simulink model "project"  (Simulink 7.6)
settings: Solver=ode45  StartTime=0.0  StopTime=10.0  RelTol=1e-3
undefined symbols (not defined in the file): des_attributefunction_support, des_figposition
libraries: simeventsgenerators1 x15, simeventssink1 x13, simeventsattributes2 x11, simeventstranslate1 x4, simeventsrouting1 x3, simeventsserver1 x1
settings Model: Creator=Tima  ModifiedByFormat=Tima  LastModifiedBy=Tima
settings SimEventsCC: propDiagAttribOutput=1  propDiagFcnCallOutput=1  propDiagStatOutput=0

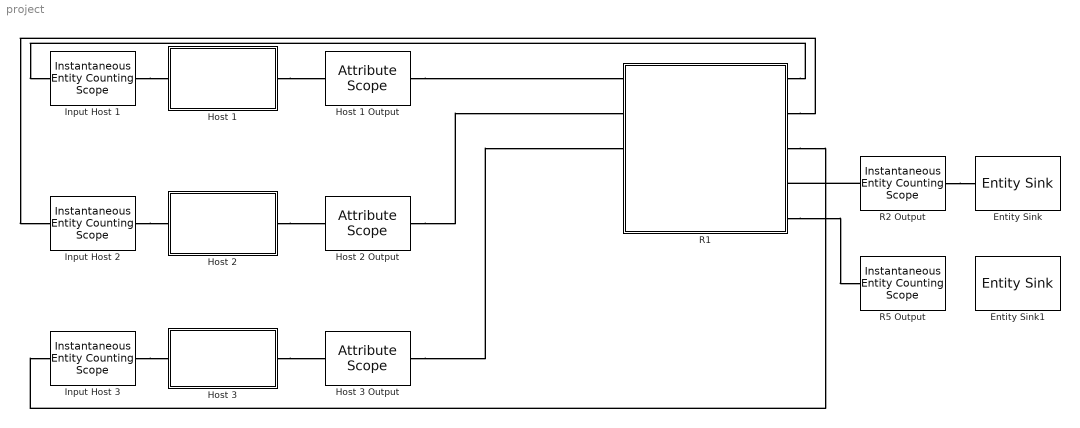
== system project ==
  Entity Sink : simeventssink1/Entity Sink  SystemSampleTime=-1  AvailableForArrivals=on  StatNumberArrived=Off
  Entity Sink1 : simeventssink1/Entity Sink  SystemSampleTime=-1  AvailableForArrivals=on  StatNumberArrived=Off
  Host 1 : Subsystem
  Host 1 Output : simeventssink1/Attribute Scope  SystemSampleTime=-1  PlotType=Stair  InputType=Attribute  NumInputs=1  AttributeNameY=dest  XInputOptionSignal=Event time  XInputOptionEntity=Event time  AttributeNameX=Count  EnableEntityOutport=on  XMin=0  XMax=10  XLimitExceededOption=Stretch axis limits  YLimitExceededOption=Stretch axis limits  AxisGrid=on  AxisLegend=off  LineDisables=""  LineColors=b  LineStyles=-  LineMarkers=.  OpenScopeAtSimStart=on  Title=""  YLabel=""  XLabel=Time  FigurePosition=des_figposition([5 25 25 25])  AxisZoom=off  DataStoreOption=Limited  DataPointsLimit=10000  StatNumberArrived=Off  ShowCountPlotted=off  ShowToolbar=on
      settings: YMin=0  YMax=10
  Host 2 : Subsystem
  Host 2 Output : simeventssink1/Attribute Scope  SystemSampleTime=-1  PlotType=Stair  InputType=Attribute  NumInputs=1  AttributeNameY=dest  XInputOptionSignal=Event time  XInputOptionEntity=Event time  AttributeNameX=Count  EnableEntityOutport=on  XMin=0  XMax=10  XLimitExceededOption=Stretch axis limits  YLimitExceededOption=Stretch axis limits  AxisGrid=on  AxisLegend=off  LineDisables=""  LineColors=b  LineStyles=-  LineMarkers=.  OpenScopeAtSimStart=on  Title=""  YLabel=""  XLabel=Time  FigurePosition=des_figposition([5 25 25 25])  AxisZoom=off  DataStoreOption=Limited  DataPointsLimit=10000  StatNumberArrived=Off  ShowCountPlotted=off  ShowToolbar=on
      settings: YMin=0  YMax=10
  Host 3 : Subsystem
  Host 3 Output : simeventssink1/Attribute Scope  SystemSampleTime=-1  PlotType=Stair  InputType=Attribute  NumInputs=1  AttributeNameY=dest  XInputOptionSignal=Event time  XInputOptionEntity=Event time  AttributeNameX=Count  EnableEntityOutport=on  XMin=0  XMax=10  XLimitExceededOption=Stretch axis limits  YLimitExceededOption=Stretch axis limits  AxisGrid=on  AxisLegend=off  LineDisables=""  LineColors=b  LineStyles=-  LineMarkers=.  OpenScopeAtSimStart=on  Title=""  YLabel=""  XLabel=Time  FigurePosition=des_figposition([5 25 25 25])  AxisZoom=off  DataStoreOption=Limited  DataPointsLimit=10000  StatNumberArrived=Off  ShowCountPlotted=off  ShowToolbar=on
      settings: YMin=0  YMax=10
  Input Host 1 : simeventssink1/Instantaneous Entity Counting Scope  SystemSampleTime=-1  PlotType=Instantaneous entity counting  InputType=Attribute  NumInputs=1  AttributeNameY=Count  XInputOptionSignal=Event time  XInputOptionEntity=Event time  AttributeNameX=Count  EnableEntityOutport=on  XMin=0  XMax=10  XLimitExceededOption=Stretch axis limits  YLimitExceededOption=Stretch axis limits  AxisGrid=on  AxisLegend=off  LineDisables=""  LineColors=b  LineStyles=-  LineMarkers=.  OpenScopeAtSimStart=on  Title=""  YLabel=Number of Entities  XLabel=Time  FigurePosition=des_figposition([5 25 25 25])  AxisZoom=off  DataStoreOption=Limited  DataPointsLimit=10000  StatNumberArrived=Off  ShowCountPlotted=off  ShowToolbar=on
      settings: YMin=0  YMax=10
  Input Host 2 : simeventssink1/Instantaneous Entity Counting Scope  SystemSampleTime=-1  PlotType=Instantaneous entity counting  InputType=Attribute  NumInputs=1  AttributeNameY=Count  XInputOptionSignal=Event time  XInputOptionEntity=Event time  AttributeNameX=Count  EnableEntityOutport=on  XMin=0  XMax=10  XLimitExceededOption=Stretch axis limits  YLimitExceededOption=Stretch axis limits  AxisGrid=on  AxisLegend=off  LineDisables=""  LineColors=b  LineStyles=-  LineMarkers=.  OpenScopeAtSimStart=on  Title=""  YLabel=Number of Entities  XLabel=Time  FigurePosition=des_figposition([5 25 25 25])  AxisZoom=off  DataStoreOption=Limited  DataPointsLimit=10000  StatNumberArrived=Off  ShowCountPlotted=off  ShowToolbar=on
      settings: YMin=0  YMax=10
  Input Host 3 : simeventssink1/Instantaneous Entity Counting Scope  SystemSampleTime=-1  PlotType=Instantaneous entity counting  InputType=Attribute  NumInputs=1  AttributeNameY=Count  XInputOptionSignal=Event time  XInputOptionEntity=Event time  AttributeNameX=Count  EnableEntityOutport=on  XMin=0  XMax=10  XLimitExceededOption=Stretch axis limits  YLimitExceededOption=Stretch axis limits  AxisGrid=on  AxisLegend=off  LineDisables=""  LineColors=b  LineStyles=-  LineMarkers=.  OpenScopeAtSimStart=on  Title=""  YLabel=Number of Entities  XLabel=Time  FigurePosition=des_figposition([5 25 25 25])  AxisZoom=off  DataStoreOption=Limited  DataPointsLimit=10000  StatNumberArrived=Off  ShowCountPlotted=off  ShowToolbar=on
      settings: YMin=0  YMax=10
  R1 : Subsystem
  R2 Output : simeventssink1/Instantaneous Entity Counting Scope  SystemSampleTime=-1  PlotType=Instantaneous entity counting  InputType=Attribute  NumInputs=1  AttributeNameY=Count  XInputOptionSignal=Event time  XInputOptionEntity=Event time  AttributeNameX=Count  EnableEntityOutport=on  XMin=0  XMax=10  XLimitExceededOption=Stretch axis limits  YLimitExceededOption=Stretch axis limits  AxisGrid=on  AxisLegend=off  LineDisables=""  LineColors=b  LineStyles=-  LineMarkers=.  OpenScopeAtSimStart=on  Title=""  YLabel=Number of Entities  XLabel=Time  FigurePosition=des_figposition([5 25 25 25])  AxisZoom=off  DataStoreOption=Limited  DataPointsLimit=10000  StatNumberArrived=Off  ShowCountPlotted=off  ShowToolbar=on
      settings: YMin=0  YMax=10
  R5 Output : simeventssink1/Instantaneous Entity Counting Scope  SystemSampleTime=-1  PlotType=Instantaneous entity counting  InputType=Attribute  NumInputs=1  AttributeNameY=Count  XInputOptionSignal=Event time  XInputOptionEntity=Event time  AttributeNameX=Count  EnableEntityOutport=on  XMin=0  XMax=10  XLimitExceededOption=Stretch axis limits  YLimitExceededOption=Stretch axis limits  AxisGrid=on  AxisLegend=off  LineDisables=""  LineColors=b  LineStyles=-  LineMarkers=.  OpenScopeAtSimStart=on  Title=""  YLabel=Number of Entities  XLabel=Time  FigurePosition=des_figposition([5 25 25 25])  AxisZoom=off  DataStoreOption=Limited  DataPointsLimit=10000  StatNumberArrived=Off  ShowCountPlotted=off  ShowToolbar=on
      settings: YMin=0  YMax=10
  connections:
  Host 1/RConn1 -- Host 1 Output/LConn1
  Host 1 Output/RConn1 -- R1/LConn1
  Host 2/RConn1 -- Host 2 Output/LConn1
  Host 2 Output/RConn1 -- R1/LConn2
  Host 3/RConn1 -- Host 3 Output/LConn1
  Host 3 Output/RConn1 -- R1/LConn3
  Input Host 3/RConn1 -- Host 3/LConn1
  R1/RConn3 -- Input Host 3/LConn1
  R1/RConn1 -- Input Host 1/LConn1
  Input Host 1/RConn1 -- Host 1/LConn1
  R1/RConn2 -- Input Host 2/LConn1
  Input Host 2/RConn1 -- Host 2/LConn1
  R2 Output/LConn1 -- R1/RConn4
  R2 Output/RConn1 -- Entity Sink/LConn1
  R1/RConn5 -- R5 Output/LConn1

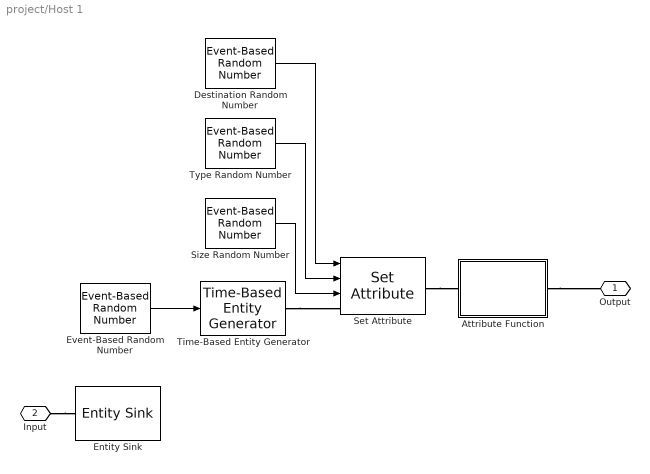
== system project/Host 1 ==
  Attribute Function : Subsystem  LoadFcn=des_attributefunction_support(gcb,'LoadFcn');  StartFcn=des_attributefunction_support(gcb,'StartFcn');  mask(Attribute Function){OutputNamePrefix=out_}
      mask prompts: OutputNamePrefix "Prefix name"
      settings: CopyFcn=des_attributefunction_support(gcb,'CopyFcn');  OpenFcn=des_attributefunction_support(gcb,'OpenFcn');  ErrorFcn=des_error_redirect
      mask Help: helpview(simeventsbhelp('attributefunction'))
      mask Display: image(des_iconLoad('attribFunction.jpg'),'center');
  Destination Random Number : simeventsgenerators1/Signal Generators/Event-Based Random Number  SystemSampleTime=-1  distribution=Discrete uniform  meanExp=1  minUnif=1  maxUnif=1  pOneBern=0.25  pSuccessBino=0.5  numTrialBino=1  meanNorm=0  stdNorm=1  minTri=1  maxTri=3  modeTri=2  thresholdLogn=0  scaleLogn=1  shapeLogn=1  pSuccessGeo=0.5  meanPoiss=1  thresholdLogl=0  scaleLogl=1  thresholdGam=0  scaleGam=1  shapeGam=1  minBeta=0  maxBeta=1  shape1Beta=1  shape2Beta=1  minUnid=1  maxUnid=6  numValueUnid=6  thresholdWbl=0  scaleWbl=1  shapeWbl=1  valueVecCont=[0 1]  cdfVecCont=[0 1]  valueVecDisc=[0 1]  probVecDisc=[0.5 0.5]  seed=897465  IsProcessed=on  isConnected=1
  Entity Sink : simeventssink1/Entity Sink  SystemSampleTime=-1  AvailableForArrivals=on  StatNumberArrived=Off
  Event-Based Random Number : simeventsgenerators1/Signal Generators/Event-Based Random Number  SystemSampleTime=-1  distribution=Poisson  meanExp=1  minUnif=1  maxUnif=1  pOneBern=0.25  pSuccessBino=0.5  numTrialBino=1  meanNorm=0  stdNorm=1  minTri=1  maxTri=3  modeTri=2  thresholdLogn=0  scaleLogn=1  shapeLogn=1  pSuccessGeo=0.5  meanPoiss=1  thresholdLogl=0  scaleLogl=1  thresholdGam=0  scaleGam=1  shapeGam=1  minBeta=0  maxBeta=1  shape1Beta=1  shape2Beta=1  minUnid=0  maxUnid=1  numValueUnid=2  thresholdWbl=0  scaleWbl=1  shapeWbl=1  valueVecCont=[0 1]  cdfVecCont=[0 1]  valueVecDisc=[0 1]  probVecDisc=[0.5 0.5]  seed=54353  IsProcessed=on  isConnected=1
  Set Attribute : simeventsattributes2/Set Attribute  DialogController=des_ddg_create  DialogControllerArgs=DataTag9  SystemSampleTime=-1  AttributeFrom=Signal port|Signal port|Signal port  AttributeName=dest|type|size  AttributeTreatAsVector=1|1|1  AttributeValue=1|1|1  AttributeCreate=on  StatNumberDeparted=Off  EvaluatedAttributeValue={[];[];[]}
  Size Random Number : simeventsgenerators1/Signal Generators/Event-Based Random Number  SystemSampleTime=-1  distribution=Discrete uniform  meanExp=1  minUnif=1  maxUnif=1  pOneBern=0.25  pSuccessBino=0.5  numTrialBino=1  meanNorm=0  stdNorm=1  minTri=1  maxTri=3  modeTri=2  thresholdLogn=0  scaleLogn=1  shapeLogn=1  pSuccessGeo=0.5  meanPoiss=1  thresholdLogl=0  scaleLogl=1  thresholdGam=0  scaleGam=1  shapeGam=1  minBeta=0  maxBeta=1  shape1Beta=1  shape2Beta=1  minUnid=1  maxUnid=2  numValueUnid=2  thresholdWbl=0  scaleWbl=1  shapeWbl=1  valueVecCont=[0 1]  cdfVecCont=[0 1]  valueVecDisc=[0 1]  probVecDisc=[0.5 0.5]  seed=79846  IsProcessed=on  isConnected=1
  Time-Based Entity Generator : simeventsgenerators1/Entity Generators/Time-Based Entity Generator  DialogController=des_ddg_create  DialogControllerArgs=DataTag11  SystemSampleTime=-1  GenerateEntitiesUpon=Intergeneration time from port t  Distribution=Constant  Minimum=0  Maximum=1  Mean=1  InitialSeed=12345  Period=1  PriorityEntityGeneration=300  GenerateEntityAtSimulationStart=on  ResponseWhenBlocked=Pause generation  ResponseWhenUnblocked=Immediate restart  EntityType=Blank  StatNumberDeparted=Off  StatPendingEntity=Off  StatAverageIntergenerationTime=Off
  Type Random Number : simeventsgenerators1/Signal Generators/Event-Based Random Number  SystemSampleTime=-1  distribution=Discrete uniform  meanExp=1  minUnif=1  maxUnif=1  pOneBern=0.25  pSuccessBino=0.5  numTrialBino=1  meanNorm=0  stdNorm=1  minTri=1  maxTri=3  modeTri=2  thresholdLogn=0  scaleLogn=1  shapeLogn=1  pSuccessGeo=0.5  meanPoiss=1  thresholdLogl=0  scaleLogl=1  thresholdGam=0  scaleGam=1  shapeGam=1  minBeta=0  maxBeta=1  shape1Beta=1  shape2Beta=1  minUnid=1  maxUnid=2  numValueUnid=2  thresholdWbl=0  scaleWbl=1  shapeWbl=1  valueVecCont=[0 1]  cdfVecCont=[0 1]  valueVecDisc=[0 1]  probVecDisc=[0.5 0.5]  seed=7865687  IsProcessed=on  isConnected=1
  Output : PMIOPort  Port=1  Side=Right
  Input : PMIOPort  Port=2  Side=Left
  wires:
  Event-Based Random Number/1 -> Time-Based Entity Generator/1
  Destination Random Number/1 -> Set Attribute/1
  Type Random Number/1 -> Set Attribute/2
  Size Random Number/1 -> Set Attribute/3
  connections:
  Set Attribute/RConn1 -- Attribute Function/LConn1
  Time-Based Entity Generator/RConn1 -- Set Attribute/LConn1
  Input/RConn1 -- Entity Sink/LConn1
  Attribute Function/RConn1 -- Output/RConn1

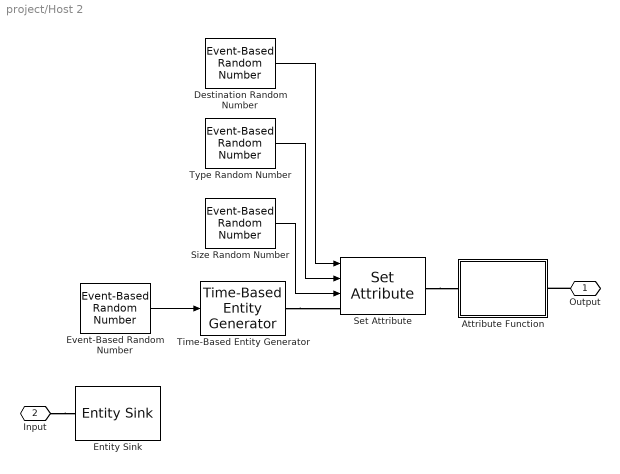
== system project/Host 2 ==
  Attribute Function : Subsystem  LoadFcn=des_attributefunction_support(gcb,'LoadFcn');  StartFcn=des_attributefunction_support(gcb,'StartFcn');  mask(Attribute Function){OutputNamePrefix=out_}
      mask prompts: OutputNamePrefix "Prefix name"
      settings: CopyFcn=des_attributefunction_support(gcb,'CopyFcn');  OpenFcn=des_attributefunction_support(gcb,'OpenFcn');  ErrorFcn=des_error_redirect
      mask Help: helpview(simeventsbhelp('attributefunction'))
      mask Display: image(des_iconLoad('attribFunction.jpg'),'center');
  Destination Random Number : simeventsgenerators1/Signal Generators/Event-Based Random Number  SystemSampleTime=-1  distribution=Discrete uniform  meanExp=1  minUnif=1  maxUnif=1  pOneBern=0.25  pSuccessBino=0.5  numTrialBino=1  meanNorm=0  stdNorm=1  minTri=1  maxTri=3  modeTri=2  thresholdLogn=0  scaleLogn=1  shapeLogn=1  pSuccessGeo=0.5  meanPoiss=1  thresholdLogl=0  scaleLogl=1  thresholdGam=0  scaleGam=1  shapeGam=1  minBeta=0  maxBeta=1  shape1Beta=1  shape2Beta=1  minUnid=1  maxUnid=6  numValueUnid=6  thresholdWbl=0  scaleWbl=1  shapeWbl=1  valueVecCont=[0 1]  cdfVecCont=[0 1]  valueVecDisc=[0 1]  probVecDisc=[0.5 0.5]  seed=8698465  IsProcessed=on  isConnected=1
  Entity Sink : simeventssink1/Entity Sink  SystemSampleTime=-1  AvailableForArrivals=on  StatNumberArrived=Off
  Event-Based Random Number : simeventsgenerators1/Signal Generators/Event-Based Random Number  SystemSampleTime=-1  distribution=Poisson  meanExp=1  minUnif=1  maxUnif=1  pOneBern=0.25  pSuccessBino=0.5  numTrialBino=1  meanNorm=0  stdNorm=1  minTri=1  maxTri=3  modeTri=2  thresholdLogn=0  scaleLogn=1  shapeLogn=1  pSuccessGeo=0.5  meanPoiss=1  thresholdLogl=0  scaleLogl=1  thresholdGam=0  scaleGam=1  shapeGam=1  minBeta=0  maxBeta=1  shape1Beta=1  shape2Beta=1  minUnid=0  maxUnid=1  numValueUnid=2  thresholdWbl=0  scaleWbl=1  shapeWbl=1  valueVecCont=[0 1]  cdfVecCont=[0 1]  valueVecDisc=[0 1]  probVecDisc=[0.5 0.5]  seed=43643  IsProcessed=on  isConnected=1
  Set Attribute : simeventsattributes2/Set Attribute  DialogController=des_ddg_create  DialogControllerArgs=DataTag20  SystemSampleTime=-1  AttributeFrom=Signal port|Signal port|Signal port  AttributeName=dest|type|size  AttributeTreatAsVector=1|1|1  AttributeValue=1|1|1  AttributeCreate=on  StatNumberDeparted=Off  EvaluatedAttributeValue={[];[];[]}
  Size Random Number : simeventsgenerators1/Signal Generators/Event-Based Random Number  SystemSampleTime=-1  distribution=Discrete uniform  meanExp=1  minUnif=1  maxUnif=1  pOneBern=0.25  pSuccessBino=0.5  numTrialBino=1  meanNorm=0  stdNorm=1  minTri=1  maxTri=3  modeTri=2  thresholdLogn=0  scaleLogn=1  shapeLogn=1  pSuccessGeo=0.5  meanPoiss=1  thresholdLogl=0  scaleLogl=1  thresholdGam=0  scaleGam=1  shapeGam=1  minBeta=0  maxBeta=1  shape1Beta=1  shape2Beta=1  minUnid=1  maxUnid=2  numValueUnid=2  thresholdWbl=0  scaleWbl=1  shapeWbl=1  valueVecCont=[0 1]  cdfVecCont=[0 1]  valueVecDisc=[0 1]  probVecDisc=[0.5 0.5]  seed=987654  IsProcessed=on  isConnected=1
  Time-Based Entity Generator : simeventsgenerators1/Entity Generators/Time-Based Entity Generator  DialogController=des_ddg_create  DialogControllerArgs=DataTag22  SystemSampleTime=-1  GenerateEntitiesUpon=Intergeneration time from port t  Distribution=Constant  Minimum=0  Maximum=1  Mean=1  InitialSeed=12345  Period=1  PriorityEntityGeneration=300  GenerateEntityAtSimulationStart=on  ResponseWhenBlocked=Pause generation  ResponseWhenUnblocked=Immediate restart  EntityType=Blank  StatNumberDeparted=Off  StatPendingEntity=Off  StatAverageIntergenerationTime=Off
  Type Random Number : simeventsgenerators1/Signal Generators/Event-Based Random Number  SystemSampleTime=-1  distribution=Discrete uniform  meanExp=1  minUnif=1  maxUnif=1  pOneBern=0.25  pSuccessBino=0.5  numTrialBino=1  meanNorm=0  stdNorm=1  minTri=1  maxTri=3  modeTri=2  thresholdLogn=0  scaleLogn=1  shapeLogn=1  pSuccessGeo=0.5  meanPoiss=1  thresholdLogl=0  scaleLogl=1  thresholdGam=0  scaleGam=1  shapeGam=1  minBeta=0  maxBeta=1  shape1Beta=1  shape2Beta=1  minUnid=1  maxUnid=2  numValueUnid=2  thresholdWbl=0  scaleWbl=1  shapeWbl=1  valueVecCont=[0 1]  cdfVecCont=[0 1]  valueVecDisc=[0 1]  probVecDisc=[0.5 0.5]  seed=869846  IsProcessed=on  isConnected=1
  Output : PMIOPort  Port=1  Side=Right
  Input : PMIOPort  Port=2  Side=Left
  wires:
  Size Random Number/1 -> Set Attribute/3
  Type Random Number/1 -> Set Attribute/2
  Destination Random Number/1 -> Set Attribute/1
  Event-Based Random Number/1 -> Time-Based Entity Generator/1
  connections:
  Input/RConn1 -- Entity Sink/LConn1
  Output/RConn1 -- Attribute Function/RConn1
  Time-Based Entity Generator/RConn1 -- Set Attribute/LConn1
  Set Attribute/RConn1 -- Attribute Function/LConn1

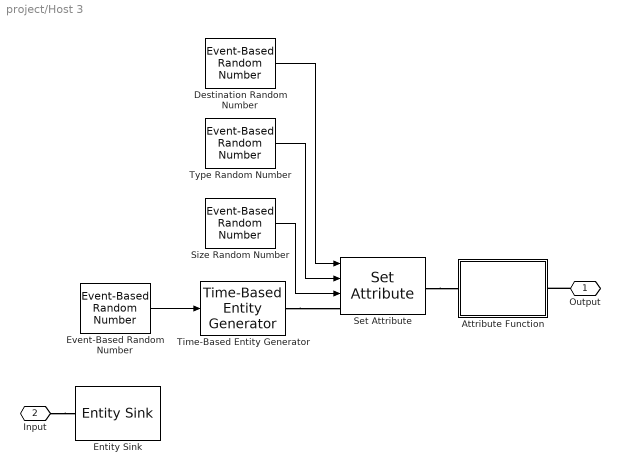
== system project/Host 3 ==
  Attribute Function : Subsystem  LoadFcn=des_attributefunction_support(gcb,'LoadFcn');  StartFcn=des_attributefunction_support(gcb,'StartFcn');  mask(Attribute Function){OutputNamePrefix=out_}
      mask prompts: OutputNamePrefix "Prefix name"
      settings: CopyFcn=des_attributefunction_support(gcb,'CopyFcn');  OpenFcn=des_attributefunction_support(gcb,'OpenFcn');  ErrorFcn=des_error_redirect
      mask Help: helpview(simeventsbhelp('attributefunction'))
      mask Display: image(des_iconLoad('attribFunction.jpg'),'center');
  Destination Random Number : simeventsgenerators1/Signal Generators/Event-Based Random Number  SystemSampleTime=-1  distribution=Discrete uniform  meanExp=1  minUnif=1  maxUnif=1  pOneBern=0.25  pSuccessBino=0.5  numTrialBino=1  meanNorm=0  stdNorm=1  minTri=1  maxTri=3  modeTri=2  thresholdLogn=0  scaleLogn=1  shapeLogn=1  pSuccessGeo=0.5  meanPoiss=1  thresholdLogl=0  scaleLogl=1  thresholdGam=0  scaleGam=1  shapeGam=1  minBeta=0  maxBeta=1  shape1Beta=1  shape2Beta=1  minUnid=1  maxUnid=6  numValueUnid=6  thresholdWbl=0  scaleWbl=1  shapeWbl=1  valueVecCont=[0 1]  cdfVecCont=[0 1]  valueVecDisc=[0 1]  probVecDisc=[0.5 0.5]  seed=964  IsProcessed=on  isConnected=1
  Entity Sink : simeventssink1/Entity Sink  SystemSampleTime=-1  AvailableForArrivals=on  StatNumberArrived=Off
  Event-Based Random Number : simeventsgenerators1/Signal Generators/Event-Based Random Number  SystemSampleTime=-1  distribution=Poisson  meanExp=1  minUnif=1  maxUnif=1  pOneBern=0.25  pSuccessBino=0.5  numTrialBino=1  meanNorm=0  stdNorm=1  minTri=1  maxTri=3  modeTri=2  thresholdLogn=0  scaleLogn=1  shapeLogn=1  pSuccessGeo=0.5  meanPoiss=1  thresholdLogl=0  scaleLogl=1  thresholdGam=0  scaleGam=1  shapeGam=1  minBeta=0  maxBeta=1  shape1Beta=1  shape2Beta=1  minUnid=0  maxUnid=1  numValueUnid=2  thresholdWbl=0  scaleWbl=1  shapeWbl=1  valueVecCont=[0 1]  cdfVecCont=[0 1]  valueVecDisc=[0 1]  probVecDisc=[0.5 0.5]  seed=12345  IsProcessed=on  isConnected=1
  Set Attribute : simeventsattributes2/Set Attribute  DialogController=des_ddg_create  DialogControllerArgs=DataTag31  SystemSampleTime=-1  AttributeFrom=Signal port|Signal port|Signal port  AttributeName=dest|type|size  AttributeTreatAsVector=1|1|1  AttributeValue=1|1|1  AttributeCreate=on  StatNumberDeparted=Off  EvaluatedAttributeValue={[];[];[]}
  Size Random Number : simeventsgenerators1/Signal Generators/Event-Based Random Number  SystemSampleTime=-1  distribution=Discrete uniform  meanExp=1  minUnif=1  maxUnif=1  pOneBern=0.25  pSuccessBino=0.5  numTrialBino=1  meanNorm=0  stdNorm=1  minTri=1  maxTri=3  modeTri=2  thresholdLogn=0  scaleLogn=1  shapeLogn=1  pSuccessGeo=0.5  meanPoiss=1  thresholdLogl=0  scaleLogl=1  thresholdGam=0  scaleGam=1  shapeGam=1  minBeta=0  maxBeta=1  shape1Beta=1  shape2Beta=1  minUnid=1  maxUnid=2  numValueUnid=2  thresholdWbl=0  scaleWbl=1  shapeWbl=1  valueVecCont=[0 1]  cdfVecCont=[0 1]  valueVecDisc=[0 1]  probVecDisc=[0.5 0.5]  seed=13245  IsProcessed=on  isConnected=1
  Time-Based Entity Generator : simeventsgenerators1/Entity Generators/Time-Based Entity Generator  DialogController=des_ddg_create  DialogControllerArgs=DataTag33  SystemSampleTime=-1  GenerateEntitiesUpon=Intergeneration time from port t  Distribution=Constant  Minimum=0  Maximum=1  Mean=1  InitialSeed=12345  Period=1  PriorityEntityGeneration=300  GenerateEntityAtSimulationStart=on  ResponseWhenBlocked=Pause generation  ResponseWhenUnblocked=Immediate restart  EntityType=Blank  StatNumberDeparted=Off  StatPendingEntity=Off  StatAverageIntergenerationTime=Off
  Type Random Number : simeventsgenerators1/Signal Generators/Event-Based Random Number  SystemSampleTime=-1  distribution=Discrete uniform  meanExp=1  minUnif=1  maxUnif=1  pOneBern=0.25  pSuccessBino=0.5  numTrialBino=1  meanNorm=0  stdNorm=1  minTri=1  maxTri=3  modeTri=2  thresholdLogn=0  scaleLogn=1  shapeLogn=1  pSuccessGeo=0.5  meanPoiss=1  thresholdLogl=0  scaleLogl=1  thresholdGam=0  scaleGam=1  shapeGam=1  minBeta=0  maxBeta=1  shape1Beta=1  shape2Beta=1  minUnid=1  maxUnid=2  numValueUnid=2  thresholdWbl=0  scaleWbl=1  shapeWbl=1  valueVecCont=[0 1]  cdfVecCont=[0 1]  valueVecDisc=[0 1]  probVecDisc=[0.5 0.5]  seed=6745  IsProcessed=on  isConnected=1
  Output : PMIOPort  Port=1  Side=Right
  Input : PMIOPort  Port=2  Side=Left
  wires:
  Event-Based Random Number/1 -> Time-Based Entity Generator/1
  Destination Random Number/1 -> Set Attribute/1
  Type Random Number/1 -> Set Attribute/2
  Size Random Number/1 -> Set Attribute/3
  connections:
  Set Attribute/RConn1 -- Attribute Function/LConn1
  Time-Based Entity Generator/RConn1 -- Set Attribute/LConn1
  Output/RConn1 -- Attribute Function/RConn1
  Input/RConn1 -- Entity Sink/LConn1

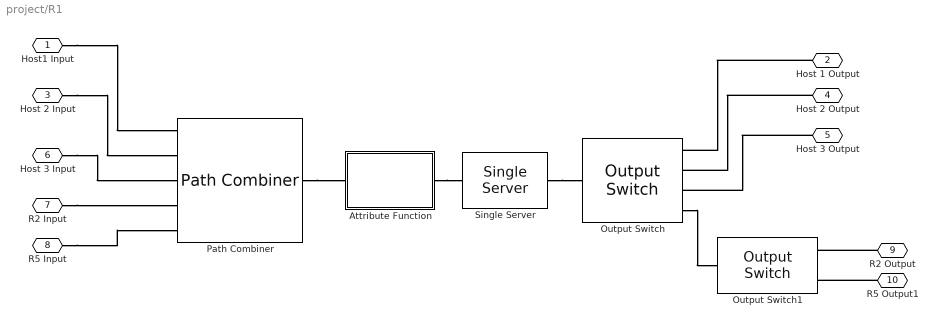
== system project/R1 ==
  Attribute Function : Subsystem  LoadFcn=des_attributefunction_support(gcb,'LoadFcn');  StartFcn=des_attributefunction_support(gcb,'StartFcn');  mask(Attribute Function){OutputNamePrefix=out_}
      mask prompts: OutputNamePrefix "Prefix name"
      settings: CopyFcn=des_attributefunction_support(gcb,'CopyFcn');  OpenFcn=des_attributefunction_support(gcb,'OpenFcn');  ErrorFcn=des_error_redirect
      mask Help: helpview(simeventsbhelp('attributefunction'))
      mask Display: image(des_iconLoad('attribFunction.jpg'),'center');
  Output Switch : simeventsrouting1/Output Switch  SystemSampleTime=-1  NumberOutputPorts=4  SwitchingCriterion=From attribute  InitialSeed=34567  AttributeName=port  InitialConditionsOpt=off  InitialConditions=1  EntityBufferOpt=off  SpecifyEventPriority=off  PriorityOutputSwitchSelectPort=4100  TimeoutPortOpt=off  StatNumberDeparted=Off  StatNumberTimedOut=Off  StatPendingEntity=Off  StatLastDeparturePort=Off  EvaluatedNumPorts=4
  Output Switch1 : simeventsrouting1/Output Switch  SystemSampleTime=-1  NumberOutputPorts=2  SwitchingCriterion=First port that is not blocked  InitialSeed=34567  AttributeName=Attribute1  InitialConditionsOpt=off  InitialConditions=1  EntityBufferOpt=off  SpecifyEventPriority=off  PriorityOutputSwitchSelectPort=4100  TimeoutPortOpt=off  StatNumberDeparted=Off  StatNumberTimedOut=Off  StatPendingEntity=Off  StatLastDeparturePort=Off  EvaluatedNumPorts=2
  Path Combiner : simeventsrouting1/Path Combiner  SystemSampleTime=-1  NumberInputPorts=5  InputPortPrecedence=IN1 port  InitialSeed=45675  SpecifyEventPriority=off  PriorityPathCombinerPortPrecedenceSelection=4100  StatNumberDeparted=Off  StatLastArrivalPort=Off  EvaluatedNumPorts=5
  Single Server : simeventsserver1/Single Server  SystemSampleTime=-1  ServiceTimeFrom=Dialog  ServiceTime=0  AttributeName=ServiceTime  PriorityServiceCompletion=500  PermitPreemption=off  SortingAttributeName=PriorityAttributeName  SortingDirection=Ascending  WriteToAttribute=off  ResidualAttributeName=ResidualServiceTime  CreateAttribute=on  EnableTOPort=off  StatNumberDeparted=Off  StatNumberInBlock=Off  StatNumberPreempted=Off  StatPendingEntity=Off  StatAverageWait=Off  StatUtilization=Off  StatNumberTimedout=Off
  Host1 Input : PMIOPort  Port=1  Side=Left
  Host 1 Output : PMIOPort  Port=2  Side=Right
  Host 2 Input : PMIOPort  Port=3  Side=Left
  Host 2 Output : PMIOPort  Port=4  Side=Right
  Host 3 Output : PMIOPort  Port=5  Side=Right
  Host 3 Input : PMIOPort  Port=6  Side=Left
  R2 Input : PMIOPort  Port=7  Side=Left
  R5 Input : PMIOPort  Port=8  Side=Left
  R2 Output : PMIOPort  Port=9  Side=Right
  R5 Output1 : PMIOPort  Port=10  Side=Right
  connections:
  Path Combiner/RConn1 -- Attribute Function/LConn1
  Host 1 Output/RConn1 -- Output Switch/RConn1
  Host 2 Output/RConn1 -- Output Switch/RConn2
  Host 3 Output/RConn1 -- Output Switch/RConn3
  Host1 Input/RConn1 -- Path Combiner/LConn1
  Host 2 Input/RConn1 -- Path Combiner/LConn2
  Host 3 Input/RConn1 -- Path Combiner/LConn3
  R2 Input/RConn1 -- Path Combiner/LConn4
  R5 Input/RConn1 -- Path Combiner/LConn5
  Output Switch/RConn4 -- Output Switch1/LConn1
  R2 Output/RConn1 -- Output Switch1/RConn1
  R5 Output1/RConn1 -- Output Switch1/RConn2
  Attribute Function/RConn1 -- Single Server/LConn1
  Single Server/RConn1 -- Output Switch/LConn1

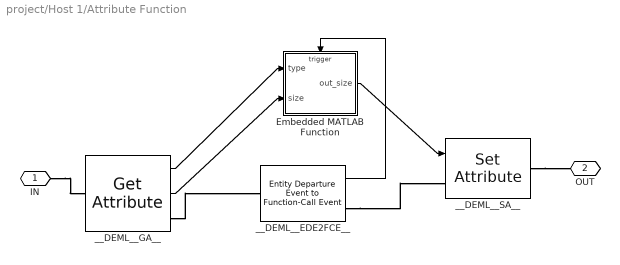
== system project/Host 1/Attribute Function ==
  Embedded MATLAB Function : Stateflow chart  TreatAsAtomicUnit=on
      settings: PropExecContextOutsideSubsystem=on
  __DEML__EDE2FCE__ : simeventstranslate1/Entity Departure Event to Function-Call Event  Priority=1  SystemSampleTime=-1  TimingFunctionCallF1=Before entity departure  EnableE1Port=off  EnableF2Port=off  TimingFunctionCallF2=Before entity departure  EnableE2Port=off  StatNumberDeparted=Off  StatNumberF1Calls=Off  StatNumberF2Calls=Off  IsInsideAFB=on
  __DEML__GA__ : simeventsattributes2/Get Attribute  Priority=1  DialogController=des_ddg_create  DialogControllerArgs=DataTag4  SystemSampleTime=-1  AttributeName=type|size  AttributeMissing=Error|Error  AttributeDefaultValue=1|1  AttributeSendTiming=Before entity departure|Before entity departure  AttributeTreatAsVector=1|1  StatNumberDeparted=Off  EvaluatedDefaultAttributeValue={[];[]}
  __DEML__SA__ : simeventsattributes2/Set Attribute  Priority=1  DialogController=des_ddg_create  DialogControllerArgs=DataTag6  SystemSampleTime=-1  AttributeFrom=Signal port  AttributeName=size  AttributeTreatAsVector=1  AttributeValue=1  AttributeCreate=on  StatNumberDeparted=Off  EvaluatedAttributeValue={[]}
  IN : PMIOPort  Port=1  Side=Left
  OUT : PMIOPort  Port=2  Side=Right
  wires:
  __DEML__EDE2FCE__/1 -> Embedded MATLAB Function/Trigger
  __DEML__GA__/1 -> Embedded MATLAB Function/1(type)
  __DEML__GA__/2 -> Embedded MATLAB Function/2(size)
  Embedded MATLAB Function/1(out_size) -> __DEML__SA__/1
  connections:
  __DEML__SA__/RConn1 -- OUT/RConn1
  IN/RConn1 -- __DEML__GA__/LConn1
  __DEML__GA__/RConn1 -- __DEML__EDE2FCE__/LConn1
  __DEML__EDE2FCE__/RConn1 -- __DEML__SA__/LConn1

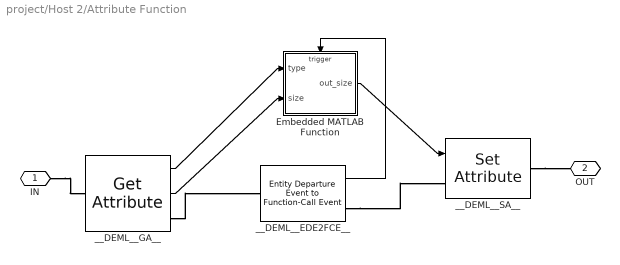
== system project/Host 2/Attribute Function ==
  Embedded MATLAB Function : Stateflow chart  TreatAsAtomicUnit=on
      settings: PropExecContextOutsideSubsystem=on
  __DEML__EDE2FCE__ : simeventstranslate1/Entity Departure Event to Function-Call Event  Priority=1  SystemSampleTime=-1  TimingFunctionCallF1=Before entity departure  EnableE1Port=off  EnableF2Port=off  TimingFunctionCallF2=Before entity departure  EnableE2Port=off  StatNumberDeparted=Off  StatNumberF1Calls=Off  StatNumberF2Calls=Off  IsInsideAFB=on
  __DEML__GA__ : simeventsattributes2/Get Attribute  Priority=1  DialogController=des_ddg_create  DialogControllerArgs=DataTag15  SystemSampleTime=-1  AttributeName=type|size  AttributeMissing=Error|Error  AttributeDefaultValue=1|1  AttributeSendTiming=Before entity departure|Before entity departure  AttributeTreatAsVector=1|1  StatNumberDeparted=Off  EvaluatedDefaultAttributeValue={[];[]}
  __DEML__SA__ : simeventsattributes2/Set Attribute  Priority=1  DialogController=des_ddg_create  DialogControllerArgs=DataTag17  SystemSampleTime=-1  AttributeFrom=Signal port  AttributeName=size  AttributeTreatAsVector=1  AttributeValue=1  AttributeCreate=on  StatNumberDeparted=Off  EvaluatedAttributeValue={[]}
  IN : PMIOPort  Port=1  Side=Left
  OUT : PMIOPort  Port=2  Side=Right
  wires:
  __DEML__EDE2FCE__/1 -> Embedded MATLAB Function/Trigger
  __DEML__GA__/1 -> Embedded MATLAB Function/1(type)
  __DEML__GA__/2 -> Embedded MATLAB Function/2(size)
  Embedded MATLAB Function/1(out_size) -> __DEML__SA__/1
  connections:
  __DEML__EDE2FCE__/RConn1 -- __DEML__SA__/LConn1
  __DEML__GA__/RConn1 -- __DEML__EDE2FCE__/LConn1
  IN/RConn1 -- __DEML__GA__/LConn1
  __DEML__SA__/RConn1 -- OUT/RConn1

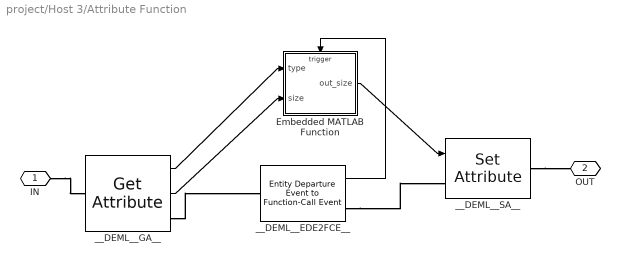
== system project/Host 3/Attribute Function ==
  Embedded MATLAB Function : Stateflow chart  TreatAsAtomicUnit=on
      settings: PropExecContextOutsideSubsystem=on
  __DEML__EDE2FCE__ : simeventstranslate1/Entity Departure Event to Function-Call Event  Priority=1  SystemSampleTime=-1  TimingFunctionCallF1=Before entity departure  EnableE1Port=off  EnableF2Port=off  TimingFunctionCallF2=Before entity departure  EnableE2Port=off  StatNumberDeparted=Off  StatNumberF1Calls=Off  StatNumberF2Calls=Off  IsInsideAFB=on
  __DEML__GA__ : simeventsattributes2/Get Attribute  Priority=1  DialogController=des_ddg_create  DialogControllerArgs=DataTag26  SystemSampleTime=-1  AttributeName=type|size  AttributeMissing=Error|Error  AttributeDefaultValue=1|1  AttributeSendTiming=Before entity departure|Before entity departure  AttributeTreatAsVector=1|1  StatNumberDeparted=Off  EvaluatedDefaultAttributeValue={[];[]}
  __DEML__SA__ : simeventsattributes2/Set Attribute  Priority=1  DialogController=des_ddg_create  DialogControllerArgs=DataTag28  SystemSampleTime=-1  AttributeFrom=Signal port  AttributeName=size  AttributeTreatAsVector=1  AttributeValue=1  AttributeCreate=on  StatNumberDeparted=Off  EvaluatedAttributeValue={[]}
  IN : PMIOPort  Port=1  Side=Left
  OUT : PMIOPort  Port=2  Side=Right
  wires:
  __DEML__EDE2FCE__/1 -> Embedded MATLAB Function/Trigger
  __DEML__GA__/1 -> Embedded MATLAB Function/1(type)
  __DEML__GA__/2 -> Embedded MATLAB Function/2(size)
  Embedded MATLAB Function/1(out_size) -> __DEML__SA__/1
  connections:
  __DEML__SA__/RConn1 -- OUT/RConn1
  IN/RConn1 -- __DEML__GA__/LConn1
  __DEML__GA__/RConn1 -- __DEML__EDE2FCE__/LConn1
  __DEML__EDE2FCE__/RConn1 -- __DEML__SA__/LConn1

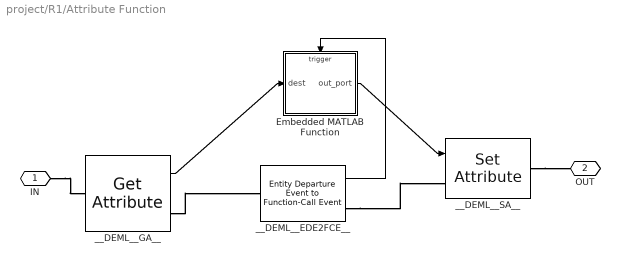
== system project/R1/Attribute Function ==
  Embedded MATLAB Function : Stateflow chart  TreatAsAtomicUnit=on
      settings: PropExecContextOutsideSubsystem=on
  __DEML__EDE2FCE__ : simeventstranslate1/Entity Departure Event to Function-Call Event  Priority=1  SystemSampleTime=-1  TimingFunctionCallF1=Before entity departure  EnableE1Port=off  EnableF2Port=off  TimingFunctionCallF2=Before entity departure  EnableE2Port=off  StatNumberDeparted=Off  StatNumberF1Calls=Off  StatNumberF2Calls=Off  IsInsideAFB=on
  __DEML__GA__ : simeventsattributes2/Get Attribute  Priority=1  DialogController=des_ddg_create  DialogControllerArgs=DataTag40  SystemSampleTime=-1  AttributeName=dest  AttributeMissing=Error  AttributeDefaultValue=1  AttributeSendTiming=Before entity departure  AttributeTreatAsVector=1  StatNumberDeparted=Off  EvaluatedDefaultAttributeValue={[]}
  __DEML__SA__ : simeventsattributes2/Set Attribute  Priority=1  DialogController=des_ddg_create  DialogControllerArgs=DataTag42  SystemSampleTime=-1  AttributeFrom=Signal port  AttributeName=port  AttributeTreatAsVector=1  AttributeValue=1  AttributeCreate=on  StatNumberDeparted=Off  EvaluatedAttributeValue={[]}
  IN : PMIOPort  Port=1  Side=Left
  OUT : PMIOPort  Port=2  Side=Right
  wires:
  __DEML__EDE2FCE__/1 -> Embedded MATLAB Function/Trigger
  __DEML__GA__/1 -> Embedded MATLAB Function/1(dest)
  Embedded MATLAB Function/1(out_port) -> __DEML__SA__/1
  connections:
  __DEML__SA__/RConn1 -- OUT/RConn1
  IN/RConn1 -- __DEML__GA__/LConn1
  __DEML__GA__/RConn1 -- __DEML__EDE2FCE__/LConn1
  __DEML__EDE2FCE__/RConn1 -- __DEML__SA__/LConn1

== matlab function Host 1/Attribute Function/Embedded MATLAB Function ==
  data: type input double; out_size output double; size input double
  events: trigger input FUNCTION_CALL_EVENT
function out_size  = fcn(type, size)
%FCN    Access and modify attributes with Embedded MATLAB Function 
% 
% Input arguments must match the attribute names.
% Output arguments must be out_<AttributeName>,
% e.g., out_ServiceTime where ServiceTime is the attribute name.
% 
% The output attribute will be created if it is not present.
%

if (type==1) 
    out_size = 512*size
else
    out_size = 256*size
end

== matlab function Host 2/Attribute Function/Embedded MATLAB Function ==
  data: type input double; out_size output double; size input double
  events: trigger input FUNCTION_CALL_EVENT
function out_size  = fcn(type, size)
%FCN    Access and modify attributes with Embedded MATLAB Function 
% 
% Input arguments must match the attribute names.
% Output arguments must be out_<AttributeName>,
% e.g., out_ServiceTime where ServiceTime is the attribute name.
% 
% The output attribute will be created if it is not present.
%

if (type==1) 
    out_size = 512*size
else
    out_size = 256*size
end

== matlab function Host 3/Attribute Function/Embedded MATLAB Function ==
  data: type input double; out_size output double; size input double
  events: trigger input FUNCTION_CALL_EVENT
function out_size  = fcn(type, size)
%FCN    Access and modify attributes with Embedded MATLAB Function 
% 
% Input arguments must match the attribute names.
% Output arguments must be out_<AttributeName>,
% e.g., out_ServiceTime where ServiceTime is the attribute name.
% 
% The output attribute will be created if it is not present.
%

if (type==1) 
    out_size = 512*size
else
    out_size = 256*size
end

== matlab function R1/Attribute Function/Embedded MATLAB Function ==
  data: dest input double; out_port output double
  events: trigger input FUNCTION_CALL_EVENT
function out_port  = fcn(dest)
%FCN    Access and modify attributes with Embedded MATLAB Function 
% 
% Input arguments must match the attribute names.
% Output arguments must be out_<AttributeName>,
% e.g., out_ServiceTime where ServiceTime is the attribute name.
% 
% The output attribute will be created if it is not present.
%


if (dest==1)
    out_port = 1
    return
end
if (dest==2)
    out_port = 2
    return
end
if (dest==3)
    out_port = 3
    return
end
out_port = 4
